simulink model "version4_lin"  (R2023b)
settings: Solver=VariableStepAuto  StartTime=0.0  StopTime=10  RelTol=1e-3
undefined symbols (not defined in the file): A_s_denom, A_s_num, c_f, C_hv_km, Cagg, Cbase1v, Cbase_hv, Cbase_mv, delta_vsc_0, G_dc_denom, G_dc_num, H_gen, H_vsm, i_d_vsc, i_q_vsc, Ibase_hv, Ibase_mv, k_d_vsm, k_p_p_vsm, k_p_q_vsm, k_vc, ki, ki_q, kp, Kp_cc, kpu, L_comp, l_f, l_grid, L_hv_km, l_t_ehvhv, l_t_hvmv, l_t_mvlv, Lagg, Lbase_hv, Lbase_mv, length_export, M_gr_denom, M_gr_num, mppt_gain, omega_nom, omega_WTR_0, omega_WTR_n, P_meas, P_t, phase_shift_test_state, phase_shifts, pie_export, Q_meas, r_f, r_grid, R_hv_km, r_sys, r_t_ehvhv, r_t_hvmv, r_t_mvlv, Ragg, Rd, rocof_slope, Rocof_test_state ... (+25)
libraries: slpidlib x9, spsFirstOrderFilterLib x1, simulink x1, spsSampleandHoldLib x1, spspowerguiLib x1
(part 2 of 3)

== system version4_lin/Subsystem ==
  v_pcc : Inport
  v_grid : Inport  Port=2
  Aggregation : Subsystem
  COllector : Subsystem
  Grid Transformer+Thevenin : Subsystem  mask{Rsource=r_grid+r_t_ehvhv, Lsource=(l_grid+l_t_ehvhv)/omega_nom}
      mask prompts: Rsource "Line resistance"; Lsource "line inductance"
      mask help:
      | RLV_NET is an 3 phase series RL with no virtual resistance termination,
      | 2 voltages as inputs and 1 current output
      mask init:
      | inv_Lsource=1/Lsource;
      mask TypeOptions Rsource: 2/Gain | 3/Gain
      mask TypeOptions Lsource: 7/Gain
  HVAC CABLE 10 PI SEGMENTS 1 : Subsystem
      settings: PortSchema="{\"entries\":[{\"content\":{\"sides\":[{\"content\":{\"connectorIds\":[\"Out2\",\"In1\",\"In2\"]},\"type\":\"ConnectorPlacement.EquallySpacedRectSide\",\"uuid\":\"364e0a5e-18fb-4479-9cea-0c32c2a31756\"},{\"content\":{\"connectorIds\":[\"Out1\",\"In3\"],\"side\":\"RIGHT\"},\"type\":\"ConnectorPlacement.EquallySpacedRectSide\",\"uuid\":\"1b6ff004-fcad-4add-afdc-525ba11bb75d\"},{\"content\":{\"side\":\"TOP\"},\"type\":\"ConnectorPlacement.EquallySpacedRectSide\",\"uuid\":\"fcc13093-d95c-447e-b2c0-1261755b0002\"}]},\"type\":\"ConnectorPlacement.EquallySpacedConnector\",\"uuid\":\"424862c2-d061-479a-b3c0-8c92e3670b7a\"}],\"packageUris\":[\"http://schema.mathworks.com/mf0/Connector/R2020b\"],\"version\":\"1.0\"}"
  Power Plant transformer : Subsystem  mask{Rsource=r_t_hvmv, Lsource=l_t_hvmv/omega_nom}
      mask prompts: Rsource "Line resistance"; Lsource "line inductance"
      mask help:
      | RLV_NET is an 3 phase series RL with no virtual resistance termination,
      | 2 voltages as inputs and 1 current output
      mask init:
      | inv_Lsource=1/Lsource;
      mask TypeOptions Rsource: 2/Gain | 3/Gain
      mask TypeOptions Lsource: 7/Gain
  "WT transformer " : Subsystem  mask{Rsource=r_t_mvlv, Lsource=l_t_mvlv/omega_nom}
      mask prompts: Rsource "Line resistance"; Lsource "line inductance"
      mask help:
      | RLV_NET is an 3 phase series RL with no virtual resistance termination,
      | 2 voltages as inputs and 1 current output
      mask init:
      | inv_Lsource=1/Lsource;
      mask TypeOptions Rsource: 2/Gain | 3/Gain
      mask TypeOptions Lsource: 7/Gain
  Output : Outport
  tag scope: omega_ref=global
  wires:
  Aggregation/2(I_HVAC_agg) -> HVAC CABLE 10 PI SEGMENTS 1/1("Isource_DQ ")
  Grid Transformer+Thevenin/1(Iline_DQ) -> Aggregation/1(I_HVAC)
  HVAC CABLE 10 PI SEGMENTS 1/2(V_L) -> Aggregation/2(V_in)
  Power Plant transformer/1(Iline_DQ) -> COllector/2(I_s), HVAC CABLE 10 PI SEGMENTS 1/3(Iinv_DQ)
  COllector/1(V_L) -> Power Plant transformer/1(Vpcc_DQ)
  COllector/2(V_R) -> "WT transformer "/2("VsDQ ")
  HVAC CABLE 10 PI SEGMENTS 1/1(V_R) -> Power Plant transformer/2("VsDQ ")
  [omega_ref] -> HVAC CABLE 10 PI SEGMENTS 1/2(omega_ref)
  [omega_ref] -> "WT transformer "/3(omega_ref)
  v_grid/1 -> Grid Transformer+Thevenin/2("VsDQ ")
  [omega_ref] -> Grid Transformer+Thevenin/3(omega_ref)
  [omega_ref] -> Power Plant transformer/3(omega_ref)
  [omega_ref] -> COllector/3(omega_ref)
  Aggregation/1(V_out) -> Grid Transformer+Thevenin/1(Vpcc_DQ)
  v_pcc/1 -> "WT transformer "/1(Vpcc_DQ)
  "WT transformer "/1(Iline_DQ) -> Output/1, COllector/1(I_L)  "i_o"
  [omega_nom] -> [omega_ref]

== system version4_lin/Subsystem1 ==
  vdq_t : Inport
  Constant : Constant  Value=v_D_t
  Constant1 : Constant  Value=v_Q_t
  Dot Product : DotProduct  OutDataTypeStr=Inherit: Inherit via internal rule
  Dot Product1 : DotProduct  OutDataTypeStr=Inherit: Inherit via internal rule
  Gain1 : Gain  Gain=v_D_t
  Gain2 : Gain  Gain=v_Q_t
  vDt : Outport
  vQt : Outport  Port=2
  wires:
  Dot Product/1 -> vDt/1
  vdq_t/1 -> Dot Product1/2, Dot Product/1
  Dot Product1/1 -> vQt/1
  Constant/1 -> Dot Product/2
  Constant1/1 -> Dot Product1/1

== system version4_lin/Subsystem2 ==
  iDQ_grid : Inport
  Constant : Constant  Value=i_d_vsc
  Constant1 : Constant  Value=i_q_vsc
  Dot Product : DotProduct  OutDataTypeStr=Inherit: Inherit via internal rule
  Dot Product1 : DotProduct  OutDataTypeStr=Inherit: Inherit via internal rule
  Gain1 : Gain  Gain=v_D_t
  Gain2 : Gain  Gain=v_Q_t
  idgrid : Outport
  iqgrid : Outport  Port=2
  wires:
  Constant1/1 -> Dot Product1/2
  Constant/1 -> Dot Product/2
  Dot Product1/1 -> iqgrid/1
  iDQ_grid/1 -> Dot Product1/1, Dot Product/1
  Dot Product/1 -> idgrid/1

== system version4_lin/Subsystem3 ==
  vDQ_vsc : Inport
  Constant : Constant  Value=v_d_vsc
  Constant1 : Constant  Value=v_q_vsc
  Dot Product : DotProduct  OutDataTypeStr=Inherit: Inherit via internal rule
  Dot Product1 : DotProduct  OutDataTypeStr=Inherit: Inherit via internal rule
  Gain1 : Gain  Gain=v_D_t
  Gain2 : Gain  Gain=v_Q_t
  vdvsc : Outport
  vqvsc : Outport  Port=2
  wires:
  Dot Product/1 -> vdvsc/1
  vDQ_vsc/1 -> Dot Product/1, Dot Product1/1
  Dot Product1/1 -> vqvsc/1
  Constant/1 -> Dot Product/2
  Constant1/1 -> Dot Product1/2

== system version4_lin/Subsystem4 ==
  V_ref_grid : Inport
  Angle ref : Inport  Port=2
  freq_ref_grid : Inport  Port=3
  Gain : Gain  Gain=2*pi
  Sum1 : Sum  Inputs=|+++
  Sum2 : Sum  Inputs=|++
  V_mag : Outport
  Angle steady state : Outport  Port=2
  omega_ref : Outport  Port=3
  wires:
  V_ref_grid/1 -> Sum2/1
  Sum1/1 -> Gain/1
  Sum2/1 -> V_mag/1
  freq_ref_grid/1 -> Sum1/1
  Gain/1 -> omega_ref/1
  Angle ref/1 -> Angle steady state/1

== system version4_lin/Subsystem5 ==
  V_ref_grid : Inport
  freq_ref_grid : Inport  Port=2
  angle_dist_grid : Inport  Port=3
  freq_dist_grid : Inport  Port=4
  V_dist_grid : Inport  Port=5
  Gain : Gain  Gain=2*pi
  Gain1 : Gain  Commented=through  Gain=1/50
  Integrator : Integrator
  Scope : Scope  NumInputPorts=2
  Sum : Sum  Inputs=|++
  Sum1 : Sum  Inputs=|+++
  grid_frequency : Constant  Value=0
  grid_voltage : Sum  Inputs=|++
  Angle : Outport
  V_mag : Outport  Port=2
  omega_ref : Outport  Port=3
  wires:
  grid_frequency/1 -> Gain1/1
  Gain1/1 -> Sum1/3
  Sum/1 -> ?
  V_ref_grid/1 -> grid_voltage/1
  Sum1/1 -> Gain/1
  V_dist_grid/1 -> grid_voltage/2, Scope/1
  grid_voltage/1 -> V_mag/1, Scope/2
  freq_ref_grid/1 -> Sum1/1
  Integrator/1 -> Sum/1
  Gain/1 -> omega_ref/1, Integrator/1
  angle_dist_grid/1 -> Angle/1
  freq_dist_grid/1 -> Sum1/2

== system version4_lin/Synchronizing torque ==
  delta_vsc : Inport
  Constant : Constant  Value=1/x_sys
  Constant1 : Constant  Value=cos(delta_vsc_0)
  Product : Product  Inputs=3
  P_grid : Outport
  wires:
  delta_vsc/1 -> Product/1
  Product/1 -> P_grid/1
  Constant/1 -> Product/2
  Constant1/1 -> Product/3

== system version4_lin/T^{-1}_vsc ==
  vtdq : Inport
  thetaPLL : Inport  Port=2
  Cos : Trigonometry  Operator=cos
  Demux1 : Demux  Outputs=2
  Display5 : Display
  Mux3 : Mux  Inputs=2
  Product{,1..3} (4 alike) : Product
  Sin : Trigonometry
  Sum : Sum  Inputs=+-
  Sum1 : Sum
  vtDQ : Outport  InitialOutput=[0,0]  VectorParamsAs1DForOutWhenUnconnected=off
  wires:
  Product3/1 -> Sum1/2
  Sum1/1 -> Mux3/2
  Demux1/1 -> Product3/1, Product/1
  vtdq/1 -> Demux1/1
  Demux1/2 -> Product2/1, Product1/1
  Sin/1 -> Product3/2, Product1/2
  Product2/1 -> Sum1/1
  Cos/1 -> Product2/2, Product/2
  Mux3/1 -> vtDQ/1, Display5/1
  thetaPLL/1 -> Cos/1, Sin/1
  Sum/1 -> Mux3/1
  Product/1 -> Sum/1
  Product1/1 -> Sum/2

== system version4_lin/T_vsc ==
  note: *
  note: =
  note: inv ([  cos(wt)   sin(wt)
      |    -sin(wt)    cos(wt)   ])
  note: [ d
      |    q ]
  note: [  al
      |     be  ]
  note: *
  note: =
  note: [  cos(wt)   -sin(wt)
      |    sin(wt)    cos(wt)   ]
  note: [ d
      |    q ]
  note: [  al
      |     be  ]
  vvscDQ : Inport
  wt : Inport  Port=2
  Cos : Trigonometry  Operator=cos
  Demux1 : Demux  Outputs=2
  Display5 : Display
  Mux3 : Mux  Inputs=2
  Product{,1..3} (4 alike) : Product
  Sin : Trigonometry
  Sum : Sum
  Sum1 : Sum  Inputs=+-
  vvscdq : Outport  InitialOutput=[0,0]  VectorParamsAs1DForOutWhenUnconnected=off
  wires:
  Demux1/1 -> Product/1, Product3/1
  wt/1 -> Sin/1, Cos/1
  Product/1 -> Sum/1
  Sum/1 -> Mux3/1
  Mux3/1 -> Display5/1, vvscdq/1
  Sum1/1 -> Mux3/2
  vvscDQ/1 -> Demux1/1
  Sin/1 -> Product1/2, Product3/2
  Product1/1 -> Sum/2
  Cos/1 -> Product/2, Product2/2
  Product2/1 -> Sum1/1
  Demux1/2 -> Product1/1, Product2/1
  Product3/1 -> Sum1/2

== system version4_lin/T_vsc1 ==
  note: [  al
      |     be  ]
  note: [ d
      |    q ]
  note: [  cos(wt)   -sin(wt)
      |    sin(wt)    cos(wt)   ]
  note: =
  note: *
  note: [  al
      |     be  ]
  note: [ d
      |    q ]
  note: inv ([  cos(wt)   sin(wt)
      |    -sin(wt)    cos(wt)   ])
  note: =
  note: *
  igDQ : Inport
  wt : Inport  Port=2
  Cos : Trigonometry  Operator=cos
  Demux1 : Demux  Outputs=2
  Display5 : Display
  Mux3 : Mux  Inputs=2
  Product{,1..3} (4 alike) : Product
  Sin : Trigonometry
  Sum : Sum
  Sum1 : Sum  Inputs=+-
  vgdq : Outport  InitialOutput=[0,0]  VectorParamsAs1DForOutWhenUnconnected=off
  wires:
  Product3/1 -> Sum1/2
  Demux1/2 -> Product2/1, Product1/1
  Product2/1 -> Sum1/1
  Cos/1 -> Product2/2, Product/2
  Product1/1 -> Sum/2
  Sin/1 -> Product3/2, Product1/2
  igDQ/1 -> Demux1/1
  Sum1/1 -> Mux3/2
  Mux3/1 -> vgdq/1, Display5/1
  Sum/1 -> Mux3/1
  Product/1 -> Sum/1
  wt/1 -> Cos/1, Sin/1
  Demux1/1 -> Product3/1, Product/1

== system version4_lin/V_dc to MSC power ==
  V_dc^2 : Inport
  V_dc_ref : Inport  Port=2
  G_dc : TransferFcn  Numerator=1*G_dc_num{1}  Denominator=G_dc_denom{1}
  Gain : Gain  Gain=1/2
  PID Controller : slpidlib/PID Controller  Controller=PI  Form=Parallel  TimeDomain=Continuous-time  UseExternalTs=off  SampleTime=-1  IntegratorMethod=Forward Euler  FilterMethod=Forward Euler  ControllerParametersSource=internal  P=20  I=5  UseKiTs=off  D=0  N=100  UseFilter=on  TunerSelectOption=Transfer Function Based (PID Tuner App)  InitialConditionSource=internal  InitialConditionForIntegrator=0  InitialConditionForFilter=0  DifferentiatorICPrevScaledInput=0  ExternalReset=none  TrackingMode=off  Kt=1  LimitOutput=off  SatLimitsSource=internal  UpperSaturationLimit=0.5  LowerSaturationLimit=-0.5  LinearizeAsGain=on  AntiWindupMode=clamping  Kb=1  LimitIntegrator=off  UpperIntegratorSaturationLimit=0.5  LowerIntegratorSaturationLimit=-0.5  POutMin=[]  POutMax=[]  IOutMin=[]  IOutMax=[]  DOutMin=[]  DOutMax=[]  NOutMin=[]  NOutMax=[]  SumOutMin=[]  SumOutMax=[]  SaturationOutMin=[]  SaturationOutMax=[]  PParamMin=[]  PParamMax=[]  IParamMin=[]  IParamMax=[]  DParamMin=[]  DParamMax=[]  NParamMin=[]  NParamMax=[]  KbParamMin=[]  KbParamMax=[]  KtParamMin=[]  KtParamMax=[]  KbOutMin=[]  KbOutMax=[]  KtOutMin=[]  KtOutMax=[]  IntegratorOutMin=[]  IntegratorOutMax=[]  FilterOutMin=[]  FilterOutMax=[]  SumI1OutMin=[]  SumI1OutMax=[]  SumI2OutMin=[]  SumI2OutMax=[]  SumI3OutMin=[]  SumI3OutMax=[]  SumI4OutMin=[]  SumI4OutMax=[]  SumDOutMin=[]  SumDOutMax=[]  DifferentiatorOutMin=[]  DifferentiatorOutMax=[]  FilterDiffOutCoefMin=[]  FilterDiffOutCoefMax=[]  ReciprocalOutMin=[]  ReciprocalOutMax=[]  SumDenOutMin=[]  SumDenOutMax=[]  SumNumOutMin=[]  SumNumOutMax=[]  DivideOutMin=[]  DivideOutMax=[]  UdiffTsProdOutMin=[]  UdiffTsProdOutMax=[]  NTsProdOutMin=[]  NTsProdOutMax=[]  UintegralTsProdOutMin=[]  UintegralTsProdOutMax=[]  UngainTsProdOutMin=[]  UngainTsProdOutMax=[]  ClampingZeroOutDataTypeStr=Inherit: Inherit via back propagation  ClampingZeroOutMin=[]  ClampingZeroOutMax=[]  FilterDenConstantOutDataTypeStr=Inherit: Inherit via back propagation  FilterDenConstantOutMin=[]  FilterDenConstantOutMax=[]  PCopyOutDataTypeStr=Inherit: Inherit via back propagation  PCopyOutMin=[]  PCopyOutMax=[]  NCopyOutDataTypeStr=Inherit: Inherit via back propagation  NCopyOutMin=[]  NCopyOutMax=[]  IntegratorContinuousStateAttributes='Delta_Pdc'  IntegratorStateMustResolveToSignalObject=off  IntegratorRTWStateStorageClass=Auto  FilterContinuousStateAttributes=''  FilterStateMustResolveToSignalObject=off  FilterRTWStateStorageClass=Auto  ParallelPVariant=InternalParameters  IdealPVariant=Disabled  IVariant=InternalParameters  DVariant=Disabled  IntegratorVariant=Continuous  SatVariant=Disabled  AWVariant=Passthrough  PCopyVariant=Disabled  TRVariant=Disabled  FdbkBlocksVariant=Forward  IdealPFdbkVariant=Disabled  SatFdbkVariant=Disabled  DerivativeFilterVariant=Disabled  NVariant=Disabled  NCopyVariant=Disabled_SignalSpec  FilterICVariant=Disabled  IntegratorICVariant=InternalICs  ExternalResetVariant=Disabled  TRSumVariant=Passthrough  SumFdbkVariant=Disabled  SumVariant=Sum_PI  TsampFilterVariant=InternalTs  TsampNgainVariant=Passthrough  TsampIntegralVariant=Disabled_SignalSpec  ExternalSaturationOutDataTypeStr=Inherit: Same as second input
  Square : Math  Commented=through  Operator=square
  Square1 : Math  Operator=square
  Sum : Sum  Inputs=|-+
  P_DC : Outport
  wires:
  V_dc^2/1 -> Square/1
  G_dc/1 -> P_DC/1
  Sum/1 -> Gain/1
  V_dc_ref/1 -> Square1/1
  Square/1 -> Sum/1
  Square1/1 -> Sum/2
  Gain/1 -> G_dc/1

== system version4_lin/V_ref generator ==
  Q_ref : Inport
  Q_vsc : Inport  Port=2
  Gain1 : Gain
  Gain3 : Gain  Gain=ki_q
  Gain9 : Gain  Gain=k_p_q_vsm
  Integrator1 : Integrator  ContinuousStateAttributes='Delta_Vdref'
  Scope : Scope  NumInputPorts=2
  Sum3 : Sum  Inputs=|-+
  Sum7 : Sum  Inputs=|+-
  Transfer Fcn : TransferFcn  Numerator=[ki_q]  Denominator=[1 ki_q]
  \Delta V^d_ref : Outport
  wires:
  Gain9/1 -> Scope/2, \Delta V^d_ref/1
  Gain1/1 -> Sum7/2
  Gain3/1 -> Integrator1/1
  Sum7/1 -> Gain3/1
  Q_ref/1 -> Sum3/2
  Q_vsc/1 -> Sum3/1
  Sum3/1 -> Sum7/1, Scope/1  "delta Q"
  Integrator1/1 -> Gain9/1, Gain1/1

== system version4_lin/VoltageControl ==
  ref : Inport
  meas : Inport  Port=2
  I filter meas : Inport  Port=3
  Constant : Constant  Value=0
  Demux1 : Demux  Outputs=[vect vect]
  Demux2 : Demux  Outputs=[vect vect]
  Demux3 : Demux  Outputs=[vect vect]
  Gain4 : Gain  Gain=c_f
  Gain5 : Gain  Gain=c_f
  Mux : Mux  Inputs=[vect vect]
  Mux1 : Mux  Inputs=3
  Mux2 : Mux  Inputs=3
  PID Controller : slpidlib/PID Controller  Commented=on  Controller=PI  Form=Parallel  TimeDomain=Continuous-time  UseExternalTs=off  SampleTime=-1  IntegratorMethod=Forward Euler  FilterMethod=Forward Euler  ControllerParametersSource=internal  P=k_vc  I=z  UseKiTs=off  D=0  N=100  UseFilter=on  TunerSelectOption=Transfer Function Based (PID Tuner App)  InitialConditionSource=internal  InitialConditionForIntegrator=0  InitialConditionForFilter=0  DifferentiatorICPrevScaledInput=0  ExternalReset=none  TrackingMode=off  Kt=1  LimitOutput=off  SatLimitsSource=internal  UpperSaturationLimit=2  LowerSaturationLimit=-2  LinearizeAsGain=off  AntiWindupMode=none  Kb=1  LimitIntegrator=off  UpperIntegratorSaturationLimit=inf  LowerIntegratorSaturationLimit=-inf  POutMin=[]  POutMax=[]  IOutMin=[]  IOutMax=[]  DOutMin=[]  DOutMax=[]  NOutMin=[]  NOutMax=[]  SumOutMin=[]  SumOutMax=[]  SaturationOutMin=[]  SaturationOutMax=[]  PParamMin=[]  PParamMax=[]  IParamMin=[]  IParamMax=[]  DParamMin=[]  DParamMax=[]  NParamMin=[]  NParamMax=[]  KbParamMin=[]  KbParamMax=[]  KtParamMin=[]  KtParamMax=[]  KbOutMin=[]  KbOutMax=[]  KtOutMin=[]  KtOutMax=[]  IntegratorOutMin=[]  IntegratorOutMax=[]  FilterOutMin=[]  FilterOutMax=[]  SumI1OutMin=[]  SumI1OutMax=[]  SumI2OutMin=[]  SumI2OutMax=[]  SumI3OutMin=[]  SumI3OutMax=[]  SumI4OutMin=[]  SumI4OutMax=[]  SumDOutMin=[]  SumDOutMax=[]  DifferentiatorOutMin=[]  DifferentiatorOutMax=[]  FilterDiffOutCoefMin=[]  FilterDiffOutCoefMax=[]  ReciprocalOutMin=[]  ReciprocalOutMax=[]  SumDenOutMin=[]  SumDenOutMax=[]  SumNumOutMin=[]  SumNumOutMax=[]  DivideOutMin=[]  DivideOutMax=[]  UdiffTsProdOutMin=[]  UdiffTsProdOutMax=[]  NTsProdOutMin=[]  NTsProdOutMax=[]  UintegralTsProdOutMin=[]  UintegralTsProdOutMax=[]  UngainTsProdOutMin=[]  UngainTsProdOutMax=[]  ClampingZeroOutDataTypeStr=Inherit: Inherit via back propagation  ClampingZeroOutMin=[]  ClampingZeroOutMax=[]  FilterDenConstantOutDataTypeStr=Inherit: Inherit via back propagation  FilterDenConstantOutMin=[]  FilterDenConstantOutMax=[]  PCopyOutDataTypeStr=Inherit: Inherit via back propagation  PCopyOutMin=[]  PCopyOutMax=[]  NCopyOutDataTypeStr=Inherit: Inherit via back propagation  NCopyOutMin=[]  NCopyOutMax=[]  IntegratorContinuousStateAttributes=''  IntegratorStateMustResolveToSignalObject=off  IntegratorRTWStateStorageClass=Auto  FilterContinuousStateAttributes=''  FilterStateMustResolveToSignalObject=off  FilterRTWStateStorageClass=Auto  ParallelPVariant=InternalParameters  IdealPVariant=Disabled  IVariant=InternalParameters  DVariant=Disabled  IntegratorVariant=Continuous  SatVariant=Disabled  AWVariant=Passthrough  PCopyVariant=Disabled  TRVariant=Disabled  FdbkBlocksVariant=Forward  IdealPFdbkVariant=Disabled  SatFdbkVariant=Disabled  DerivativeFilterVariant=Disabled  NVariant=Disabled  NCopyVariant=Disabled_SignalSpec  FilterICVariant=Disabled  IntegratorICVariant=InternalICs  ExternalResetVariant=Disabled  TRSumVariant=Passthrough  SumFdbkVariant=Disabled  SumVariant=Sum_PI  TsampFilterVariant=InternalTs  TsampNgainVariant=Passthrough  TsampIntegralVariant=Disabled_SignalSpec  ExternalSaturationOutDataTypeStr=Inherit: Same as second input
  PID Controller1 : slpidlib/PID Controller  Commented=on  Controller=PI  Form=Ideal  TimeDomain=Continuous-time  UseExternalTs=off  SampleTime=-1  IntegratorMethod=Forward Euler  FilterMethod=Forward Euler  ControllerParametersSource=internal  P=k_vc  I=z  UseKiTs=off  D=0  N=100  UseFilter=on  TunerSelectOption=Transfer Function Based (PID Tuner App)  InitialConditionSource=internal  InitialConditionForIntegrator=0  InitialConditionForFilter=0  DifferentiatorICPrevScaledInput=0  ExternalReset=none  TrackingMode=off  Kt=1  LimitOutput=off  SatLimitsSource=internal  UpperSaturationLimit=2  LowerSaturationLimit=-2  LinearizeAsGain=off  AntiWindupMode=none  Kb=1  LimitIntegrator=off  UpperIntegratorSaturationLimit=inf  LowerIntegratorSaturationLimit=-inf  POutMin=[]  POutMax=[]  IOutMin=[]  IOutMax=[]  DOutMin=[]  DOutMax=[]  NOutMin=[]  NOutMax=[]  SumOutMin=[]  SumOutMax=[]  SaturationOutMin=[]  SaturationOutMax=[]  PParamMin=[]  PParamMax=[]  IParamMin=[]  IParamMax=[]  DParamMin=[]  DParamMax=[]  NParamMin=[]  NParamMax=[]  KbParamMin=[]  KbParamMax=[]  KtParamMin=[]  KtParamMax=[]  KbOutMin=[]  KbOutMax=[]  KtOutMin=[]  KtOutMax=[]  IntegratorOutMin=[]  IntegratorOutMax=[]  FilterOutMin=[]  FilterOutMax=[]  SumI1OutMin=[]  SumI1OutMax=[]  SumI2OutMin=[]  SumI2OutMax=[]  SumI3OutMin=[]  SumI3OutMax=[]  SumI4OutMin=[]  SumI4OutMax=[]  SumDOutMin=[]  SumDOutMax=[]  DifferentiatorOutMin=[]  DifferentiatorOutMax=[]  FilterDiffOutCoefMin=[]  FilterDiffOutCoefMax=[]  ReciprocalOutMin=[]  ReciprocalOutMax=[]  SumDenOutMin=[]  SumDenOutMax=[]  SumNumOutMin=[]  SumNumOutMax=[]  DivideOutMin=[]  DivideOutMax=[]  UdiffTsProdOutMin=[]  UdiffTsProdOutMax=[]  NTsProdOutMin=[]  NTsProdOutMax=[]  UintegralTsProdOutMin=[]  UintegralTsProdOutMax=[]  UngainTsProdOutMin=[]  UngainTsProdOutMax=[]  ClampingZeroOutDataTypeStr=Inherit: Inherit via back propagation  ClampingZeroOutMin=[]  ClampingZeroOutMax=[]  FilterDenConstantOutDataTypeStr=Inherit: Inherit via back propagation  FilterDenConstantOutMin=[]  FilterDenConstantOutMax=[]  PCopyOutDataTypeStr=Inherit: Inherit via back propagation  PCopyOutMin=[]  PCopyOutMax=[]  NCopyOutDataTypeStr=Inherit: Inherit via back propagation  NCopyOutMin=[]  NCopyOutMax=[]  IntegratorContinuousStateAttributes=''  IntegratorStateMustResolveToSignalObject=off  IntegratorRTWStateStorageClass=Auto  FilterContinuousStateAttributes=''  FilterStateMustResolveToSignalObject=off  FilterRTWStateStorageClass=Auto  ParallelPVariant=Passthrough  IdealPVariant=InternalParameters  IVariant=InternalParameters  DVariant=Disabled  IntegratorVariant=Continuous  SatVariant=Disabled  AWVariant=Passthrough  PCopyVariant=Disabled  TRVariant=Disabled  FdbkBlocksVariant=Forward  IdealPFdbkVariant=Disabled  SatFdbkVariant=Disabled  DerivativeFilterVariant=Disabled  NVariant=Disabled  NCopyVariant=Disabled_SignalSpec  FilterICVariant=Disabled  IntegratorICVariant=InternalICs  ExternalResetVariant=Disabled  TRSumVariant=Passthrough  SumFdbkVariant=Disabled  SumVariant=Sum_PI  TsampFilterVariant=InternalTs  TsampNgainVariant=Passthrough  TsampIntegralVariant=Disabled_SignalSpec  ExternalSaturationOutDataTypeStr=Inherit: Same as second input
  PID Controller2 : slpidlib/PID Controller  Controller=PI  Form=Ideal  TimeDomain=Continuous-time  UseExternalTs=off  SampleTime=-1  IntegratorMethod=Forward Euler  FilterMethod=Forward Euler  ControllerParametersSource=internal  P=kpu  I=1/Tnu  UseKiTs=off  D=0  N=100  UseFilter=on  TunerSelectOption=Transfer Function Based (PID Tuner App)  InitialConditionSource=internal  InitialConditionForIntegrator=0  InitialConditionForFilter=0  DifferentiatorICPrevScaledInput=0  ExternalReset=none  TrackingMode=off  Kt=1  LimitOutput=off  SatLimitsSource=internal  UpperSaturationLimit=2  LowerSaturationLimit=-2  LinearizeAsGain=off  AntiWindupMode=none  Kb=1  LimitIntegrator=off  UpperIntegratorSaturationLimit=inf  LowerIntegratorSaturationLimit=-inf  POutMin=[]  POutMax=[]  IOutMin=[]  IOutMax=[]  DOutMin=[]  DOutMax=[]  NOutMin=[]  NOutMax=[]  SumOutMin=[]  SumOutMax=[]  SaturationOutMin=[]  SaturationOutMax=[]  PParamMin=[]  PParamMax=[]  IParamMin=[]  IParamMax=[]  DParamMin=[]  DParamMax=[]  NParamMin=[]  NParamMax=[]  KbParamMin=[]  KbParamMax=[]  KtParamMin=[]  KtParamMax=[]  KbOutMin=[]  KbOutMax=[]  KtOutMin=[]  KtOutMax=[]  IntegratorOutMin=[]  IntegratorOutMax=[]  FilterOutMin=[]  FilterOutMax=[]  SumI1OutMin=[]  SumI1OutMax=[]  SumI2OutMin=[]  SumI2OutMax=[]  SumI3OutMin=[]  SumI3OutMax=[]  SumI4OutMin=[]  SumI4OutMax=[]  SumDOutMin=[]  SumDOutMax=[]  DifferentiatorOutMin=[]  DifferentiatorOutMax=[]  FilterDiffOutCoefMin=[]  FilterDiffOutCoefMax=[]  ReciprocalOutMin=[]  ReciprocalOutMax=[]  SumDenOutMin=[]  SumDenOutMax=[]  SumNumOutMin=[]  SumNumOutMax=[]  DivideOutMin=[]  DivideOutMax=[]  UdiffTsProdOutMin=[]  UdiffTsProdOutMax=[]  NTsProdOutMin=[]  NTsProdOutMax=[]  UintegralTsProdOutMin=[]  UintegralTsProdOutMax=[]  UngainTsProdOutMin=[]  UngainTsProdOutMax=[]  ClampingZeroOutDataTypeStr=Inherit: Inherit via back propagation  ClampingZeroOutMin=[]  ClampingZeroOutMax=[]  FilterDenConstantOutDataTypeStr=Inherit: Inherit via back propagation  FilterDenConstantOutMin=[]  FilterDenConstantOutMax=[]  PCopyOutDataTypeStr=Inherit: Inherit via back propagation  PCopyOutMin=[]  PCopyOutMax=[]  NCopyOutDataTypeStr=Inherit: Inherit via back propagation  NCopyOutMin=[]  NCopyOutMax=[]  IntegratorContinuousStateAttributes='Delta_i_ref_d'  IntegratorStateMustResolveToSignalObject=off  IntegratorRTWStateStorageClass=Auto  FilterContinuousStateAttributes=''  FilterStateMustResolveToSignalObject=off  FilterRTWStateStorageClass=Auto  ParallelPVariant=Passthrough  IdealPVariant=InternalParameters  IVariant=InternalParameters  DVariant=Disabled  IntegratorVariant=Continuous  SatVariant=Disabled  AWVariant=Passthrough  PCopyVariant=Disabled  TRVariant=Disabled  FdbkBlocksVariant=Forward  IdealPFdbkVariant=Disabled  SatFdbkVariant=Disabled  DerivativeFilterVariant=Disabled  NVariant=Disabled  NCopyVariant=Disabled_SignalSpec  FilterICVariant=Disabled  IntegratorICVariant=InternalICs  ExternalResetVariant=Disabled  TRSumVariant=Passthrough  SumFdbkVariant=Disabled  SumVariant=Sum_PI  TsampFilterVariant=InternalTs  TsampNgainVariant=Passthrough  TsampIntegralVariant=Disabled_SignalSpec  ExternalSaturationOutDataTypeStr=Inherit: Same as second input
  PID Controller4 : slpidlib/PID Controller  Controller=PI  Form=Ideal  TimeDomain=Continuous-time  UseExternalTs=off  SampleTime=-1  IntegratorMethod=Forward Euler  FilterMethod=Forward Euler  ControllerParametersSource=internal  P=kpu  I=1/Tnu  UseKiTs=off  D=0  N=100  UseFilter=on  TunerSelectOption=Transfer Function Based (PID Tuner App)  InitialConditionSource=internal  InitialConditionForIntegrator=0  InitialConditionForFilter=0  DifferentiatorICPrevScaledInput=0  ExternalReset=none  TrackingMode=off  Kt=1  LimitOutput=off  SatLimitsSource=internal  UpperSaturationLimit=2  LowerSaturationLimit=-2  LinearizeAsGain=off  AntiWindupMode=none  Kb=1  LimitIntegrator=off  UpperIntegratorSaturationLimit=inf  LowerIntegratorSaturationLimit=-inf  POutMin=[]  POutMax=[]  IOutMin=[]  IOutMax=[]  DOutMin=[]  DOutMax=[]  NOutMin=[]  NOutMax=[]  SumOutMin=[]  SumOutMax=[]  SaturationOutMin=[]  SaturationOutMax=[]  PParamMin=[]  PParamMax=[]  IParamMin=[]  IParamMax=[]  DParamMin=[]  DParamMax=[]  NParamMin=[]  NParamMax=[]  KbParamMin=[]  KbParamMax=[]  KtParamMin=[]  KtParamMax=[]  KbOutMin=[]  KbOutMax=[]  KtOutMin=[]  KtOutMax=[]  IntegratorOutMin=[]  IntegratorOutMax=[]  FilterOutMin=[]  FilterOutMax=[]  SumI1OutMin=[]  SumI1OutMax=[]  SumI2OutMin=[]  SumI2OutMax=[]  SumI3OutMin=[]  SumI3OutMax=[]  SumI4OutMin=[]  SumI4OutMax=[]  SumDOutMin=[]  SumDOutMax=[]  DifferentiatorOutMin=[]  DifferentiatorOutMax=[]  FilterDiffOutCoefMin=[]  FilterDiffOutCoefMax=[]  ReciprocalOutMin=[]  ReciprocalOutMax=[]  SumDenOutMin=[]  SumDenOutMax=[]  SumNumOutMin=[]  SumNumOutMax=[]  DivideOutMin=[]  DivideOutMax=[]  UdiffTsProdOutMin=[]  UdiffTsProdOutMax=[]  NTsProdOutMin=[]  NTsProdOutMax=[]  UintegralTsProdOutMin=[]  UintegralTsProdOutMax=[]  UngainTsProdOutMin=[]  UngainTsProdOutMax=[]  ClampingZeroOutDataTypeStr=Inherit: Inherit via back propagation  ClampingZeroOutMin=[]  ClampingZeroOutMax=[]  FilterDenConstantOutDataTypeStr=Inherit: Inherit via back propagation  FilterDenConstantOutMin=[]  FilterDenConstantOutMax=[]  PCopyOutDataTypeStr=Inherit: Inherit via back propagation  PCopyOutMin=[]  PCopyOutMax=[]  NCopyOutDataTypeStr=Inherit: Inherit via back propagation  NCopyOutMin=[]  NCopyOutMax=[]  IntegratorContinuousStateAttributes='Delta_i_ref_d'  IntegratorStateMustResolveToSignalObject=off  IntegratorRTWStateStorageClass=Auto  FilterContinuousStateAttributes=''  FilterStateMustResolveToSignalObject=off  FilterRTWStateStorageClass=Auto  ParallelPVariant=Passthrough  IdealPVariant=InternalParameters  IVariant=InternalParameters  DVariant=Disabled  IntegratorVariant=Continuous  SatVariant=Disabled  AWVariant=Passthrough  PCopyVariant=Disabled  TRVariant=Disabled  FdbkBlocksVariant=Forward  IdealPFdbkVariant=Disabled  SatFdbkVariant=Disabled  DerivativeFilterVariant=Disabled  NVariant=Disabled  NCopyVariant=Disabled_SignalSpec  FilterICVariant=Disabled  IntegratorICVariant=InternalICs  ExternalResetVariant=Disabled  TRSumVariant=Passthrough  SumFdbkVariant=Disabled  SumVariant=Sum_PI  TsampFilterVariant=InternalTs  TsampNgainVariant=Passthrough  TsampIntegralVariant=Disabled_SignalSpec  ExternalSaturationOutDataTypeStr=Inherit: Same as second input
  Sum1 : Sum  Inputs=|+-
  Sum2 : Sum  Inputs=+-|
  Sum4 : Sum  Inputs=++-
  Sum5 : Sum  Inputs=+++
  Transfer Fcn2 : TransferFcn  Commented=on  Denominator=[0.005 1]
  Transfer Fcn3 : TransferFcn  Commented=on  Denominator=[0.005 1]
  d-axis v control : Scope  NumInputPorts=3
  q-axis v control : Scope  NumInputPorts=3
  I_ref_unsat : Outport
  wires:
  Mux2/1 -> d-axis v control/2
  Transfer Fcn2/1 -> Sum5/3, Mux1/1
  PID Controller4/1 -> Mux2/2, Sum4/2
  Mux1/1 -> q-axis v control/2
  Demux3/2 -> Sum2/1
  meas/1 -> Demux1/1
  Gain5/1 -> Mux1/3, Sum5/1
  PID Controller2/1 -> Sum5/2, Mux1/2
  Demux2/2 -> Transfer Fcn2/1
  Sum5/1 -> Mux/2, q-axis v control/3
  Mux/1 -> I_ref_unsat/1
  Gain4/1 -> Mux2/3, Sum4/3
  Demux1/2 -> Gain4/1, Sum2/2
  Sum1/1 -> PID Controller4/1, d-axis v control/1
  Demux1/1 -> Sum1/2, Gain5/1
  ref/1 -> Demux3/1
  Sum2/1 -> PID Controller2/1, q-axis v control/1
  Transfer Fcn3/1 -> Mux2/1, Sum4/1
  Demux2/1 -> Transfer Fcn3/1
  I filter meas/1 -> Demux2/1
  Sum4/1 -> Mux/1, d-axis v control/3
  Demux3/1 -> Sum1/1

== system version4_lin/WT transformer  ==
  note: Network
  note: VIRTUAL RESITANCE
  Vpcc_DQ : Inport
  "VsDQ " : Inport  Port=2
  omega_ref : Inport  Port=3
  1 : Gain  Gain=inv_Lsource
  2 : Gain  Gain=Rsource
  3 : Gain  Gain=Rsource
  4 : Gain  Gain=inv_Lsource
  7 : Gain  Gain=Lsource
  Demux1 : Demux  Outputs=2
  Demux2 : Demux  Outputs=2
  Id : Scope
  Iline_D_int : Integrator  UpperSaturationLimit=50  LowerSaturationLimit=-1000  ContinuousStateAttributes='Delta_i_vsc_D'
  Iline_Q_int : Integrator  UpperSaturationLimit=50  LowerSaturationLimit=-1000  ContinuousStateAttributes='Delta_i_vsc_Q'
  Iq : Scope
  Mux1 : Mux  Inputs=2
  Mux4 : Mux  Inputs=2
  Product1 : Product
  Product2 : Product
  Sum1 : Sum  Inputs=|+---
  Sum8 : Sum  Inputs=|+-+-
  Iline_DQ : Outport  VectorParamsAs1DForOutWhenUnconnected=off
  wires:
  7/1 -> [wL]
  [Vpcc_Q] -> Sum1/1
  [Vpcc_D] -> Sum8/1
  Demux2/1 -> Mux4/1, [Vpcc_D]
  Demux2/2 -> Mux4/2, [Vpcc_Q]
  Sum1/1 -> 4/1
  1/1 -> Iline_D_int/1
  Iline_D_int/1 -> Product1/2, Id/1, 2/1, Mux1/1
  Iline_Q_int/1 -> Mux1/2, Iq/1, Product2/2, 3/1
  Sum8/1 -> 1/1
  2/1 -> Sum8/4
  Product2/1 -> Sum8/3
  3/1 -> Sum1/4
  4/1 -> Iline_Q_int/1
  Product1/1 -> Sum1/3
  [wL] -> Product1/1, Product2/1
  Demux1/1 -> Sum8/2
  Demux1/2 -> Sum1/2
  "VsDQ "/1 -> Demux1/1
  Vpcc_DQ/1 -> Demux2/1
  Mux1/1 -> Iline_DQ/1
  omega_ref/1 -> 7/1

== system version4_lin/WT transformer 1 ==
  note: Network
  note: VIRTUAL RESITANCE
  Vpcc_DQ : Inport
  "VsDQ " : Inport  Port=2
  omega_ref : Inport  Port=3
  1 : Gain  Gain=inv_Lsource
  2 : Gain  Gain=Rsource
  3 : Gain  Gain=Rsource
  4 : Gain  Gain=inv_Lsource
  7 : Gain  Gain=Lsource
  Demux1 : Demux  Outputs=2
  Demux2 : Demux  Outputs=2
  Id : Scope
  Iline_D_int : Integrator  UpperSaturationLimit=50  LowerSaturationLimit=-1000  ContinuousStateAttributes='Delta_i_grid_D'
  Iline_Q_int : Integrator  UpperSaturationLimit=50  LowerSaturationLimit=-1000  ContinuousStateAttributes='Delta_i_grid_Q'
  Iq : Scope
  Mux1 : Mux  Inputs=2
  Mux4 : Mux  Inputs=2
  Product1 : Product
  Product2 : Product
  Sum1 : Sum  Inputs=|+---
  Sum8 : Sum  Inputs=|+-+-
  Iline_DQ : Outport  VectorParamsAs1DForOutWhenUnconnected=off
  wires:
  7/1 -> [wL]
  [Vpcc_Q] -> Sum1/1
  [Vpcc_D] -> Sum8/1
  Demux2/1 -> Mux4/1, [Vpcc_D]
  Demux2/2 -> Mux4/2, [Vpcc_Q]
  Sum1/1 -> 4/1
  1/1 -> Iline_D_int/1
  Iline_D_int/1 -> Product1/2, Id/1, 2/1, Mux1/1
  Iline_Q_int/1 -> Mux1/2, Iq/1, Product2/2, 3/1
  Sum8/1 -> 1/1
  2/1 -> Sum8/4
  Product2/1 -> Sum8/3
  3/1 -> Sum1/4
  4/1 -> Iline_Q_int/1
  Product1/1 -> Sum1/3
  [wL] -> Product1/1, Product2/1
  Demux1/1 -> Sum8/2
  Demux1/2 -> Sum1/2
  "VsDQ "/1 -> Demux1/1
  Vpcc_DQ/1 -> Demux2/1
  Mux1/1 -> Iline_DQ/1
  omega_ref/1 -> 7/1

== system version4_lin/gen->rotor ==
  Tgen : Inport
  Gain : Gain  Gain=1/(2*H_gen)
  Integrator : Integrator  ContinuousStateAttributes='Delta_omega_gen'
  Sum : Sum  Inputs=+-|
  Sum1 : Sum  Inputs=|+-
  Transfer Fcn : TransferFcn  Commented=on  Numerator=M_gr_num{1}  Denominator=M_gr_denom{1}  ContinuousStateAttributes="{\"Delta_torque_shaft\", \"Delta_torque_WTR\"}"
  gen_to_wtr : TransferFcn  Numerator=wwtr_over_wgen_num{1}  Denominator=wwtr_over_wgen_denom{1}  ContinuousStateAttributes="\"Delta_omega_WTR\""
  to_Tshaft : TransferFcn  Numerator=A_s_num{1}  Denominator=A_s_denom{1}  ContinuousStateAttributes="\"Delta_Tshaft\""
  omega_gen : Outport
  wires:
  Sum/1 -> Gain/1
  Gain/1 -> Integrator/1
  Tgen/1 -> Sum/2
  Transfer Fcn/1 -> ?
  gen_to_wtr/1 -> Sum1/1
  Integrator/1 -> Sum1/2, gen_to_wtr/1, omega_gen/1
  Sum1/1 -> to_Tshaft/1
  to_Tshaft/1 -> Sum/1

== system version4_lin/modulator ==
  v_dc : Inport
  v_m : Inport  Port=2
  Constant : Constant  Value=[v_D0_t; v_Q0_t]
  Constant1 : Constant  Value=0.9999
  Gain : Gain  Gain=1/(sqrt(3/2))
  Gain1 : Gain  Gain=1/2
  Product : Product
  Product1 : Product
  Sum : Sum  Inputs=|++
  Out1 : Outport
  wires:
  Gain/1 -> Out1/1
  Constant/1 -> Product/1
  v_dc/1 -> Gain1/1
  Sum/1 -> Gain/1
  Product/1 -> Sum/2
  v_m/1 -> Product1/1
  Product1/1 -> Sum/1
  Constant1/1 -> Product1/2
  Gain1/1 -> Product/2

== system version4_lin/mppt ==
  note: Remember to add SI->PU conversion before output
  omega_gen : Inport
  Gain : Gain  Gain=omega_WTR_n
  Gain1 : Gain  Gain=1/(15e6)
  MPPT_GAIN : Gain  Gain=mppt_gain
  P_ref : Outport
  wires:
  omega_gen/1 -> Gain/1
  MPPT_GAIN/1 -> Gain1/1
  Gain/1 -> MPPT_GAIN/1
  Gain1/1 -> P_ref/1

== system version4_lin/msc_power to T_gen ==
  P_gen : Inport
  Divide : Product  Inputs=*/
  turbine omega operating point : Constant  Value=(omega_WTR_0/omega_WTR_n)
  Tgen : Outport
  wires:
  P_gen/1 -> Divide/1
  turbine omega operating point/1 -> Divide/2
  Divide/1 -> Tgen/1

== system version4_lin/omega and theta grid ==
  oemga_grid : Inport
  phase grid dist : Inport  Port=2
  Sum9 : Sum  Inputs=|-+
  omega_nom : Constant  Value=0
  wpsl1 : Integrator  UpperSaturationLimit=300  LowerSaturationLimit=-100
  Out1 : Outport
  wires:
  wpsl1/1 -> Out1/1
  omega_nom/1 -> Sum9/1
  oemga_grid/1 -> Sum9/2
  Sum9/1 -> wpsl1/1

== system version4_lin/omega turbine to T_gen ==
  omega_WTR : Inport
  Constant : Constant  Value=P_t
  Divide : Product  Inputs=**/
  Square : Math  Operator=square
  turbine omega operating point : Constant  Value=(omega_WTR_0/omega_WTR_n)
  Tgen : Outport
  wires:
  omega_WTR/1 -> Divide/1
  Divide/1 -> Tgen/1
  Constant/1 -> Divide/2
  turbine omega operating point/1 -> Square/1
  Square/1 -> Divide/3

== system version4_lin/theta_ref generator ==
  P_ref : Inport
  P_vsc : Inport  Port=2
  Constant : Constant  Value=0.59*180/pi
  Gain1 : Gain  Gain=1/(2*pi)
  Gain2 : Gain  Gain=omega_nom
  Gain3 : Gain  Gain=1/(2*H_vsm)
  Gain6 : Gain  Commented=through  Gain=k_p_p_vsm
  Gain7 : Gain  Gain=180/pi
  Gain8 : Gain  Gain=k_d_vsm
  Integrator : Integrator  WrappedStateUpperValue=2*pi  WrappedStateLowerValue=0  ContinuousStateAttributes='Delta_theta_rad'
  Integrator1 : Integrator  ContinuousStateAttributes="\"Delta_omega_ref\""
  Mux : Mux  Inputs=2
  Sum : Sum  Inputs=|++
  Sum1 : Sum  Inputs=+-|
  Sum6 : Sum  Inputs=++|
  Sum7 : Sum  Inputs=|+-
  Transfer Fcn : TransferFcn  Denominator=[2*H_vsm k_d_vsm]  ContinuousStateAttributes='Delta_omega'
  vsm : Scope  NumInputPorts=3
  \Delta_theta_vsm : Outport
  wires:
  Gain3/1 -> Integrator1/1
  Sum1/1 -> Sum7/1, vsm/1  "delta P"
  Gain8/1 -> Sum7/2
  Gain6/1 -> Gain2/1  "Delta_omega"
  Sum7/1 -> Gain3/1  "delta P"
  Gain2/1 -> Sum6/2, Gain1/1
  P_ref/1 -> Mux/1, Sum1/1
  P_vsc/1 -> Mux/2, Sum1/2
  Integrator/1 -> Gain7/1, \Delta_theta_vsm/1  "theta_ref_rad"
  Sum6/1 -> Integrator/1  "omega_ref"
  Mux/1 -> ?
  Gain1/1 -> vsm/2  "Frequency"
  Sum/1 -> vsm/3  "theta_ref_deg"
  Gain7/1 -> Sum/1  "theta_ref_deg"
  Constant/1 -> Sum/2
  Integrator1/1 -> Gain8/1, Gain6/1

== system version4_lin/Subsystem/Aggregation ==
  I_HVAC : Inport
  V_in : Inport  Port=2
  Demux1 : Demux  Outputs=[vect vect]
  Demux2 : Demux  Outputs=2
  Gain2 : Gain  Gain=1/(1*vect)
  Gain3 : Gain  Gain=ones(vect,1)
  Gain4 : Gain  Gain=ones(vect,1)
  Mux2 : Mux  Inputs=2
  Mux3 : Mux  Inputs=2
  Sum of Elements : Sum  Inputs=+
  Sum of Elements1 : Sum  Inputs=+
  V_out : Outport
  I_HVAC_agg : Outport  Port=2
  wires:
  Mux3/1 -> Gain2/1
  Gain3/1 -> Mux2/1
  Demux2/1 -> Gain3/1
  Sum of Elements1/1 -> Mux3/2
  Gain4/1 -> Mux2/2
  Demux2/2 -> Gain4/1
  Sum of Elements/1 -> Mux3/1
  Gain2/1 -> I_HVAC_agg/1
  V_in/1 -> Demux2/1
  Mux2/1 -> V_out/1
  I_HVAC/1 -> Demux1/1
  Demux1/1 -> Sum of Elements/1
  Demux1/2 -> Sum of Elements1/1

== system version4_lin/Subsystem/COllector ==
  I_L : Inport
  I_s : Inport  Port=2
  omega_ref : Inport  Port=3
  Gain2 : Gain  Commented=through  Gain=1/Vbase_mv
  Gain3 : Gain  Commented=through  Gain=1/Vbase_mv
  Gain4 : Gain  Commented=through  Gain=Ibase_mv
  Gain5 : Gain  Commented=through  Gain=Ibase_mv
  Scope : Scope  NumInputPorts=2
  collector : Subsystem  mask{Rsource=Ragg/Zbase_mv, Csource=(Cagg/Cbase_mv)/omega_nom, Lsource=(Lagg/Lbase_mv)/omega_nom}
      mask prompts: Rsource "Series R"; Csource "Net Capacitance"; Lsource "Net Inductance"
      mask help:
      | PI network, capacitance to enter is total.
      | Left and right current as input. Left and right voltage as output
      mask init:
      | inv_Csource=2/Csource;
      | inv_Lsource=1/Lsource;
      mask TypeOptions Rsource: 2/Gain | 3/Gain
      mask TypeOptions Csource: 8/Gain
      mask TypeOptions Lsource: 7/Gain
  V_L : Outport
  V_R : Outport  Port=2
  wires:
  Gain4/1 -> collector/1(Iload_DQ)
  collector/1(VpccR_DQ) -> Gain2/1
  Gain2/1 -> V_R/1
  collector/2(VpccL_DQ) -> Gain3/1
  I_s/1 -> Gain5/1
  Gain3/1 -> Scope/1, V_L/1
  Gain5/1 -> collector/2("Isource_DQ ")
  I_L/1 -> Scope/2, Gain4/1
  omega_ref/1 -> collector/3(omega_ref)

== system version4_lin/Subsystem/Grid Transformer+Thevenin ==
  note: Network
  note: VIRTUAL RESITANCE
  Vpcc_DQ : Inport
  "VsDQ " : Inport  Port=2
  omega_ref : Inport  Port=3
  1 : Gain  Gain=inv_Lsource
  2 : Gain  Gain=Rsource
  3 : Gain  Gain=Rsource
  4 : Gain  Gain=inv_Lsource
  7 : Gain  Gain=Lsource
  Demux1 : Demux  Outputs=2
  Demux2 : Demux  Outputs=2
  Id : Scope
  Iline_D_int : Integrator  UpperSaturationLimit=50  LowerSaturationLimit=-1000
  Iline_Q_int : Integrator  UpperSaturationLimit=50  LowerSaturationLimit=-1000
  Iq : Scope
  Mux1 : Mux  Inputs=2
  Mux4 : Mux  Inputs=2
  Product1 : Product
  Product2 : Product
  Sum1 : Sum  Inputs=|+---
  Sum8 : Sum  Inputs=|+-+-
  Iline_DQ : Outport  VectorParamsAs1DForOutWhenUnconnected=off
  wires:
  7/1 -> [wL]
  omega_ref/1 -> 7/1
  [Vpcc_Q] -> Sum1/1
  [Vpcc_D] -> Sum8/1
  Demux2/1 -> Mux4/1, [Vpcc_D]
  Demux2/2 -> Mux4/2, [Vpcc_Q]
  Sum1/1 -> 4/1
  1/1 -> Iline_D_int/1
  Iline_D_int/1 -> Product1/2, Id/1, 2/1, Mux1/1
  Iline_Q_int/1 -> Mux1/2, Iq/1, Product2/2, 3/1
  Sum8/1 -> 1/1
  2/1 -> Sum8/4
  Product2/1 -> Sum8/3
  3/1 -> Sum1/4
  4/1 -> Iline_Q_int/1
  Product1/1 -> Sum1/3
  [wL] -> Product1/1, Product2/1
  Demux1/1 -> Sum8/2
  Demux1/2 -> Sum1/2
  "VsDQ "/1 -> Demux1/1
  Vpcc_DQ/1 -> Demux2/1
  Mux1/1 -> Iline_DQ/1

== system version4_lin/Subsystem/HVAC CABLE 10 PI SEGMENTS 1 ==
  "Isource_DQ " : Inport
  omega_ref : Inport  Port=2
  Iinv_DQ : Inport  Port=3
  Gain1 : Gain  Commented=through  Gain=1/Vbase_hv
  Gain2 : Gain  Commented=through  Gain=1/Vbase_hv
  Gain4 : Gain  Commented=through  Gain=Ibase_hv
  Gain5 : Gain  Commented=through  Gain=Ibase_hv
  Goto : Goto  Commented=on  GotoTag=omega_ref
  RC sys1 : Subsystem  mask{Csource=(C_hv_km*length_export/pie_export/2/Cbase_hv)/omega_nom, Rd=0.0001, VD0=0, VQ0=0}
      mask prompts: Csource "Net Capacitance"; Rd "Rdamp"
      mask help:
      | PI network, capacitance to enter is total.
      | Left and right current as input. Left and right voltage as output
      mask init:
      | inv_Csource=1/Csource;
      mask TypeOptions Csource: 8/Gain
      mask TypeOptions Rd: 1/Gain | 2/Gain
      mask TypeOptions VD0: VcpdR_int/InitialCondition
      mask TypeOptions VQ0: VcpqR_int/InitialCondition
  RLC_NET 11 : Subsystem  mask{Csource=(C_hv_km*length_export/pie_export/Cbase_hv)/omega_nom, Rsource=(R_hv_km*length_export/pie_export)/Zbase_hv, Lsource=(L_hv_km*length_export/pie_export/Lbase_hv)/omega_nom}
      mask prompts: Csource "line capacitance 1 side"; Rsource "Line resistance"; Lsource "line inductance"
      mask help:
      | RL with C terminations on right,
      | Left Voltage  and Right current input, Right voltage and left current output
      mask init:
      | inv_Csource=1/Csource;
      | inv_Lsource=1/Lsource;
      mask TypeOptions Csource: 8/Gain
      mask TypeOptions Rsource: 2/Gain | 3/Gain
      mask TypeOptions Lsource: 7/Gain
  RLC_NET 12 : Subsystem  mask{Csource=(C_hv_km*length_export/pie_export/Cbase_hv)/omega_nom, Rsource=(R_hv_km*length_export/pie_export)/Zbase_hv, Lsource=(L_hv_km*length_export/pie_export/Lbase_hv)/omega_nom}
      mask prompts: Csource "line capacitance 1 side"; Rsource "Line resistance"; Lsource "line inductance"
      mask help:
      | RL with C terminations on right,
      | Left Voltage  and Right current input, Right voltage and left current output
      mask init:
      | inv_Csource=1/Csource;
      | inv_Lsource=1/Lsource;
      mask TypeOptions Csource: 8/Gain
      mask TypeOptions Rsource: 2/Gain | 3/Gain
      mask TypeOptions Lsource: 7/Gain
  RLC_NET 13 : Subsystem  mask{Csource=(C_hv_km*length_export/pie_export/Cbase_hv)/omega_nom, Rsource=(R_hv_km*length_export/pie_export)/Zbase_hv, Lsource=(L_hv_km*length_export/pie_export/Lbase_hv)/omega_nom}
      mask prompts: Csource "line capacitance 1 side"; Rsource "Line resistance"; Lsource "line inductance"
      mask help:
      | RL with C terminations on right,
      | Left Voltage  and Right current input, Right voltage and left current output
      mask init:
      | inv_Csource=1/Csource;
      | inv_Lsource=1/Lsource;
      mask TypeOptions Csource: 8/Gain
      mask TypeOptions Rsource: 2/Gain | 3/Gain
      mask TypeOptions Lsource: 7/Gain
  RLC_NET 14 : Subsystem  mask{Csource=(C_hv_km*length_export/pie_export/Cbase_hv)/omega_nom, Rsource=(R_hv_km*length_export/pie_export)/Zbase_hv, Lsource=(L_hv_km*length_export/pie_export/Lbase_hv)/omega_nom}
      mask prompts: Csource "line capacitance 1 side"; Rsource "Line resistance"; Lsource "line inductance"
      mask help:
      | RL with C terminations on right,
      | Left Voltage  and Right current input, Right voltage and left current output
      mask init:
      | inv_Csource=1/Csource;
      | inv_Lsource=1/Lsource;
      mask TypeOptions Csource: 8/Gain
      mask TypeOptions Rsource: 2/Gain | 3/Gain
      mask TypeOptions Lsource: 7/Gain
  RLC_NET 15 : Subsystem  mask{Csource=(C_hv_km*length_export/pie_export/Cbase_hv)/omega_nom, Rsource=(R_hv_km*length_export/pie_export)/Zbase_hv, Lsource=(L_hv_km*length_export/pie_export/Lbase_hv)/omega_nom}
      mask prompts: Csource "line capacitance 1 side"; Rsource "Line resistance"; Lsource "line inductance"
      mask help:
      | RL with C terminations on right,
      | Left Voltage  and Right current input, Right voltage and left current output
      mask init:
      | inv_Csource=1/Csource;
      | inv_Lsource=1/Lsource;
      mask TypeOptions Csource: 8/Gain
      mask TypeOptions Rsource: 2/Gain | 3/Gain
      mask TypeOptions Lsource: 7/Gain
  RLC_NET 16 : Subsystem  mask{Csource=(C_hv_km*length_export/pie_export/Cbase_hv)/omega_nom, Rsource=(R_hv_km*length_export/pie_export)/Zbase_hv, Lsource=(L_hv_km*length_export/pie_export/Lbase_hv)/omega_nom}
      mask prompts: Csource "line capacitance 1 side"; Rsource "Line resistance"; Lsource "line inductance"
      mask help:
      | RL with C terminations on right,
      | Left Voltage  and Right current input, Right voltage and left current output
      mask init:
      | inv_Csource=1/Csource;
      | inv_Lsource=1/Lsource;
      mask TypeOptions Csource: 8/Gain
      mask TypeOptions Rsource: 2/Gain | 3/Gain
      mask TypeOptions Lsource: 7/Gain
  RLC_NET 17 : Subsystem  mask{Csource=(C_hv_km*length_export/pie_export/Cbase_hv)/omega_nom, Rsource=(R_hv_km*length_export/pie_export)/Zbase_hv, Lsource=(L_hv_km*length_export/pie_export/Lbase_hv)/omega_nom}
      mask prompts: Csource "line capacitance 1 side"; Rsource "Line resistance"; Lsource "line inductance"
      mask help:
      | RL with C terminations on right,
      | Left Voltage  and Right current input, Right voltage and left current output
      mask init:
      | inv_Csource=1/Csource;
      | inv_Lsource=1/Lsource;
      mask TypeOptions Csource: 8/Gain
      mask TypeOptions Rsource: 2/Gain | 3/Gain
      mask TypeOptions Lsource: 7/Gain
  RLC_NET 18 : Subsystem  mask{Csource=(C_hv_km*length_export/pie_export/Cbase_hv)/omega_nom, Rsource=(R_hv_km*length_export/pie_export)/Zbase_hv, Lsource=(L_hv_km*length_export/pie_export/Lbase_hv)/omega_nom}
      mask prompts: Csource "line capacitance 1 side"; Rsource "Line resistance"; Lsource "line inductance"
      mask help:
      | RL with C terminations on right,
      | Left Voltage  and Right current input, Right voltage and left current output
      mask init:
      | inv_Csource=1/Csource;
      | inv_Lsource=1/Lsource;
      mask TypeOptions Csource: 8/Gain
      mask TypeOptions Rsource: 2/Gain | 3/Gain
      mask TypeOptions Lsource: 7/Gain
  RLC_NET 19 : Subsystem  mask{Csource=(C_hv_km*length_export/pie_export/Cbase_hv)/omega_nom, Rsource=(R_hv_km*length_export/pie_export)/Zbase_hv, Lsource=(L_hv_km*length_export/pie_export/Lbase_hv)/omega_nom}
      mask prompts: Csource "line capacitance 1 side"; Rsource "Line resistance"; Lsource "line inductance"
      mask help:
      | RL with C terminations on right,
      | Left Voltage  and Right current input, Right voltage and left current output
      mask init:
      | inv_Csource=1/Csource;
      | inv_Lsource=1/Lsource;
      mask TypeOptions Csource: 8/Gain
      mask TypeOptions Rsource: 2/Gain | 3/Gain
      mask TypeOptions Lsource: 7/Gain
  RLC_NET 20 : Subsystem  mask{Csource=(C_hv_km*length_export/pie_export/2/Cbase_hv)/omega_nom, Rsource=(R_hv_km*length_export/pie_export)/Zbase_hv, Lsource=(L_hv_km*length_export/pie_export/Lbase_hv)/omega_nom}
      mask prompts: Csource "line capacitance 1 side"; Rsource "Line resistance"; Lsource "line inductance"
      mask help:
      | RL with C terminations on right,
      | Left Voltage  and Right current input, Right voltage and left current output
      mask init:
      | inv_Csource=1/Csource;
      | inv_Lsource=1/Lsource;
      mask TypeOptions Csource: 8/Gain
      mask TypeOptions Rsource: 2/Gain | 3/Gain
      mask TypeOptions Lsource: 7/Gain
  RLV_NET 1 : Subsystem  mask{Rsource=0, Lsource=(L_comp/Lbase_hv)/omega_nom}
      mask prompts: Rsource "Line resistance"; Lsource "line inductance"
      mask help:
      | RLV_NET is an 3 phase series RL with no virtual resistance termination,
      | 2 voltages as inputs and 1 current output
      mask init:
      | inv_Lsource=1/Lsource;
      mask TypeOptions Rsource: 2/Gain | 3/Gain
      mask TypeOptions Lsource: 7/Gain
  RLV_NET 2 : Subsystem  mask{Rsource=0, Lsource=(L_comp/Lbase_hv)/omega_nom}
      mask prompts: Rsource "Line resistance"; Lsource "line inductance"
      mask help:
      | RLV_NET is an 3 phase series RL with no virtual resistance termination,
      | 2 voltages as inputs and 1 current output
      mask init:
      | inv_Lsource=1/Lsource;
      mask TypeOptions Rsource: 2/Gain | 3/Gain
      mask TypeOptions Lsource: 7/Gain
  Sum2 : Sum  Inputs=++|
  Sum3 : Sum  Inputs=-+|
  V_R : Outport
  V_L : Outport  Port=2
  wires:
  RC sys1/1(VpccR_DQ) -> Gain1/1, RLV_NET 1/1(Vpcc_DQ), RLC_NET 11/2("VsDQ ")
  Gain1/1 -> V_L/1
  "Isource_DQ "/1 -> Gain4/1
  RLC_NET 11/1(Iline_DQ) -> RC sys1/1(Iload_DQ)
  Sum2/1 -> RC sys1/2("Isource_DQ ")
  Gain4/1 -> Sum2/2
  RLV_NET 1/1(Iline_DQ) -> Sum2/1
  omega_ref/1 -> Goto/1
  [omega_ref] -> RLC_NET 11/3(omega_ref)
  [omega_ref] -> RLC_NET 12/3(omega_ref)
  [omega_ref] -> RLC_NET 14/3(omega_ref)
  [omega_ref] -> RLC_NET 13/3(omega_ref)
  [omega_ref] -> RLC_NET 15/3(omega_ref)
  [omega_ref] -> RLC_NET 20/3(omega_ref)
  [omega_ref] -> RLC_NET 18/3(omega_ref)
  [omega_ref] -> RLC_NET 19/3(omega_ref)
  [omega_ref] -> RLC_NET 16/3(omega_ref)
  [omega_ref] -> RLC_NET 17/3(omega_ref)
  Iinv_DQ/1 -> Gain5/1
  Gain2/1 -> V_R/1
  RLC_NET 20/2(Vpcc_DQ) -> RLV_NET 2/1(Vpcc_DQ), Gain2/1
  Gain5/1 -> Sum3/2
  RLV_NET 2/1(Iline_DQ) -> Sum3/1
  [omega_ref] -> RLV_NET 2/2(omega_ref)
  RLC_NET 11/2(Vpcc_DQ) -> RLC_NET 12/2("VsDQ ")
  RLC_NET 12/1(Iline_DQ) -> RLC_NET 11/1(Iinv_DQ)
  RLC_NET 13/1(Iline_DQ) -> RLC_NET 12/1(Iinv_DQ)
  RLC_NET 12/2(Vpcc_DQ) -> RLC_NET 13/2("VsDQ ")
  RLC_NET 13/2(Vpcc_DQ) -> RLC_NET 14/2("VsDQ ")
  RLC_NET 14/1(Iline_DQ) -> RLC_NET 13/1(Iinv_DQ)
  RLC_NET 14/2(Vpcc_DQ) -> RLC_NET 15/2("VsDQ ")
  RLC_NET 15/1(Iline_DQ) -> RLC_NET 14/1(Iinv_DQ)
  RLC_NET 16/1(Iline_DQ) -> RLC_NET 15/1(Iinv_DQ)
  RLC_NET 17/1(Iline_DQ) -> RLC_NET 16/1(Iinv_DQ)
  RLC_NET 18/1(Iline_DQ) -> RLC_NET 17/1(Iinv_DQ)
  RLC_NET 16/2(Vpcc_DQ) -> RLC_NET 17/2("VsDQ ")
  RLC_NET 15/2(Vpcc_DQ) -> RLC_NET 16/2("VsDQ ")
  RLC_NET 19/1(Iline_DQ) -> RLC_NET 18/1(Iinv_DQ)
  RLC_NET 18/2(Vpcc_DQ) -> RLC_NET 19/2("VsDQ ")
  RLC_NET 17/2(Vpcc_DQ) -> RLC_NET 18/2("VsDQ ")
  RLC_NET 19/2(Vpcc_DQ) -> RLC_NET 20/2("VsDQ ")
  RLC_NET 20/1(Iline_DQ) -> RLC_NET 19/1(Iinv_DQ)
  Sum3/1 -> RLC_NET 20/1(Iinv_DQ)
  [omega_ref] -> RLV_NET 1/2(omega_ref), RC sys1/3(omega_ref)
